simulink model "synchronous"  (Simulink 7.3)
settings: Solver=ode45  StartTime=0.0  StopTime=.1  RelTol=1e-3
libraries: powerlib x11
settings Model: Creator=USRE  LastModifiedBy=USRE

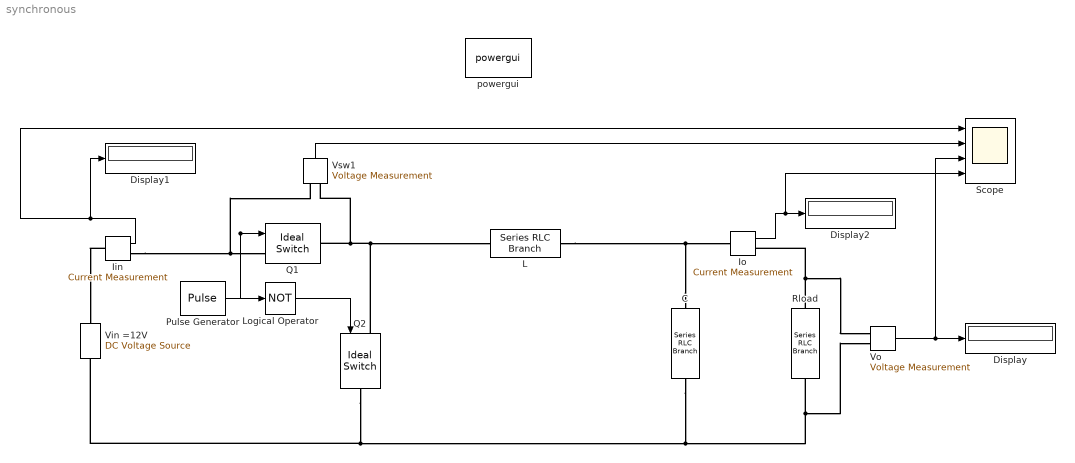
== system synchronous ==
  C : powerlib/Elements/Series RLC Branch  DialogController=POWERSYS.PowerSysDialog  PhysicalDomain=powersysdomain  SubClassName=unknown  LeftPortType=p1  RightPortType=p1  LConnTagsString=__new0  RConnTagsString=__new0  BranchType=C  Resistance=0.1  Inductance=1e-3  SetiL0=off  InitialCurrent=0  Capacitance=120e-6  Setx0=off  InitialVoltage=0  Measurements=Branch voltage
  Display : Display
  Display1 : Display
  Display2 : Display
  Iin : powerlib/Measurements/Current Measurement  DialogController=POWERSYS.PowerSysDialog  SystemSampleTime=-1  PhasorSimulation=off  OutputType=Complex  PSBequivalent=0
  Io : powerlib/Measurements/Current Measurement  DialogController=POWERSYS.PowerSysDialog  SystemSampleTime=-1  PhasorSimulation=off  OutputType=Complex  PSBequivalent=0
  L : powerlib/Elements/Series RLC Branch  DialogController=POWERSYS.PowerSysDialog  PhysicalDomain=powersysdomain  SubClassName=unknown  LeftPortType=p1  RightPortType=p1  LConnTagsString=__new0  RConnTagsString=__new0  BranchType=L  Resistance=1  Inductance=11.5e-6  SetiL0=off  InitialCurrent=0  Capacitance=1e-6  Setx0=off  InitialVoltage=0  Measurements=None
  Logical Operator : Logic  Operator=NOT  AllPortsSameDT=off  OutDataTypeMode=boolean  LogicDataType=fixdt(0, 8)  OutDataTypeStr=boolean
  Pulse Generator : DiscretePulseGenerator  PulseType=Time based  Amplitude=1  Period=1/(100e3)  PulseWidth=50  PhaseDelay=0  SampleTime=1
  Q1 : powerlib/Power Electronics/Ideal Switch  DialogController=POWERSYS.PowerSysDialog  SystemSampleTime=-1  Ron=0.001  Lon=0  IC=0  Rs=1e5  Cs=inf  Measurements=off
  Q2 : powerlib/Power Electronics/Ideal Switch  DialogController=POWERSYS.PowerSysDialog  SystemSampleTime=-1  Ron=0.001  Lon=0  IC=0  Rs=1e5  Cs=inf  Measurements=off
  Rload : powerlib/Elements/Series RLC Branch  DialogController=POWERSYS.PowerSysDialog  PhysicalDomain=powersysdomain  SubClassName=unknown  LeftPortType=p1  RightPortType=p1  LConnTagsString=__new0  RConnTagsString=__new0  BranchType=R  Resistance=2  Inductance=1e-3  SetiL0=off  InitialCurrent=0  Capacitance=150e-6  Setx0=off  InitialVoltage=0  Measurements=Branch voltage
  Scope : Scope  NumInputPorts=4
      settings: TimeRange=2.375478927332895e-010  YMin=2.49939~0~-5~-5  YMax=2.4994~3~5~5
  Vin =12V : powerlib/Electrical Sources/DC Voltage Source  DialogController=POWERSYS.PowerSysDialog  SystemSampleTime=-1  Amplitude=12  Measurements=None
  Vo : powerlib/Measurements/Voltage Measurement  DialogController=POWERSYS.PowerSysDialog  SystemSampleTime=-1  PhasorSimulation=off  OutputType=Complex  PSBequivalent=0
  Vsw1 : powerlib/Measurements/Voltage Measurement  DialogController=POWERSYS.PowerSysDialog  SystemSampleTime=-1  PhasorSimulation=off  OutputType=Complex  PSBequivalent=0
  powergui : powerlib/powergui  Priority=1  SystemSampleTime=-1  SimulationMode=Continuous  SampleTime=50e-6  frequency=60  SPID=off  DisableSnubberDevices=off  DisableRonSwitches=off  DisableVfSwitches=off  SwTol=0  Interpol=off  frequencyindice=0  echomessages=off  HookPort=off  DisplayEquations=off  FunctionMessages=off  EnableUseOfTLC=off  x0status=blocks  RestoreLinks=warning  Frange=[0:2:500]  Ylog=off  Xlog=on  ShowGrid=off  save=off  variable=ZData  ZoomFFT=on  StartTime=0.0  cycles=1  DisplayStyle=1  fundamental=60  FreqAxis=off  MaxFrequency=1000  frequencyindicesteady=1  RmsSteady=1  display=off  Ts=0  methode=off
  wires:
  Vo/1 -> Display/1, Scope/3
  Io/1 -> Display2/1, Scope/4
  Iin/1 -> Display1/1, Scope/1
  Pulse Generator/1 -> Q1/1, Logical Operator/1
  Logical Operator/1 -> Q2/1
  Vsw1/1 -> Scope/2
  connections:
  Q2/LConn1 -- L/LConn1 -- Q1/RConn1 -- Vsw1/LConn2
  Rload/LConn1 -- Io/RConn1 -- Vo/LConn1
  C/LConn1 -- L/RConn1 -- Io/LConn1
  Rload/RConn1 -- Q2/RConn1 -- Vin =12V/LConn1 -- C/RConn1 -- Vo/LConn2
  Iin/RConn1 -- Q1/LConn1 -- Vsw1/LConn1
  Iin/LConn1 -- Vin =12V/RConn1
